simulink model "quadcopter_dynamic_model"  (R2016b)
settings: Solver=FixedStepAuto  StartTime=0.0  StopTime=30  FixedStep=0.001  MaxStep=0.004  RelTol=1e-3
PreLoadFcn:
  | init
undefined symbols (not defined in the file or in its folder): Data, Data_SL_Info, W, X, Y, Z
libraries: robotlib x7
settings Model: Creator=ADAM  LastModifiedBy=consti
settings SolverCC: ExtrapolationOrder=1
settings DataIOCC: MaxDataPoints=1  SaveFormat=Structure  SignalLoggingSaveFormat=ModelDataLogs  SaveOutput=off  SignalLogging=off  DSMLogging=off  SaveTime=off  OutputSaveName=model_out  SignalLoggingName=model_out
settings OptimizationCC: ExpressionDepthLimit=2147483647  LifeSpan=inf  SimCompilerOptimization=on
settings DebuggingCC: UnderspecifiedInitializationDetection=Classic  MergeDetectMultiDrivingBlocksExec=none  InheritedTsInSrcMsg=none  MultiTaskDSMMsg=warning  MultiTaskCondExecSysMsg=none  UnconnectedInputMsg=none  UnconnectedOutputMsg=none  UnconnectedLineMsg=none  StateNameClashWarn=warning  SFUnexpectedBacktrackingDiag=warning  SFNoUnconditionalDefaultTransitionDiag=warning  SFExecutionAtInitializationDiag=none
settings HardwareCC: ProdBitPerPointer=32  ProdBitPerSizeT=32  ProdBitPerPtrDiffT=32  ProdLargestAtomicFloat=None  ProdWordSize=32  ProdHWDeviceType=Generic->32-bit x86 compatible
settings ModelReferenceCC: UpdateModelReferenceTargets=IfOutOfDate  PropagateSignalLabelsOutOfModel=off
settings CodeAppCC: MaxIdLength=95
settings GRTTargetCC: TargetLangStandard=C89/C90 (ANSI)  GeneratePreprocessorConditionals=Disable all
settings ConfigComp: CovMetricSettings=dw  CovHtmlReporting=on  CovSaveCumulativeToWorkspaceVar=on  CovSaveSingleToWorkspaceVar=on  CovExternalEMLEnable=off  CovSFcnEnable=off

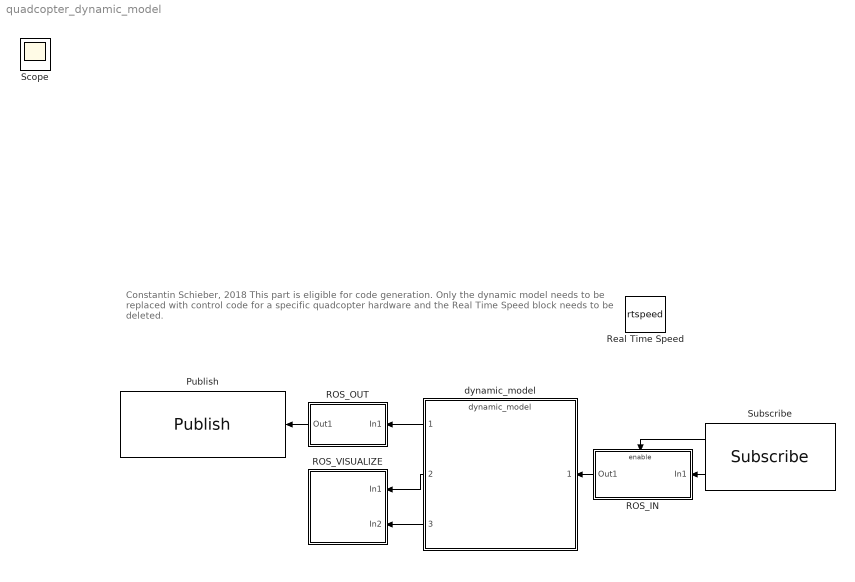
== system quadcopter_dynamic_model ==
  note: Constantin Schieber, 2018
      |
      | This part is eligible for code generation. Only the dynamic model needs to be replaced with control code
      | for a specific quadcopter hardware and the Real Time Speed block needs to be deleted.
  Publish : robotlib/Publish  SourceLibraryInfo=This block requires Robotics System Toolbox  topicSource=Specify your own  topic=/dyn_model_measurments  messageType=std_msgs/Float32MultiArray  messageQueueLength=1
  ROS_IN : Subsystem
  ROS_OUT : Subsystem
  ROS_VISUALIZE : Subsystem
  Real Time Speed : S-Function  FunctionName=rtspeed  Parameters=speed  SFunctionDeploymentMode=off  EnableBusSupport=off  mask(Simulink Realtime Synchronization){speed=1}
      mask prompts: speed "Simulation Speed (1 = realtime)"
      mask help: Slows down simulation to desired real time speed.
      mask Display:
      | ang=(0:0.0125:1)*2*pi;
      | xp=100*cos(ang);
      | yp=100*sin(ang);
      | plot(-145,-130,155,170,xp,yp,[0 0 70*sqrt(2)/2],[70 0 70*sqrt(2)/2],[-40 40 40 -40 -40],[150 150 120 120 150],[-15 -15],[120 98.5],[15 15],[120 98.5],[100*cos((45+9)/180*pi) 100*cos((45+9)/180*pi)+30 100*cos((45-9)/180*pi)+30 100*cos((45-9)/180*pi)],[100*sin((45+9)/180*pi) 100*sin((45+9)/180*pi)+30 100*sin((45-9)/180*pi)+30 100*sin((45-9)/180*pi)]);
  Subscribe : robotlib/Subscribe  SourceLibraryInfo=This block requires Robotics System Toolbox  topicSource=Specify your own  topic=/control_system_pwm  messageType=std_msgs/Float32MultiArray  sampleTime=-1  messageQueueLength=1
  dynamic_model : ModelReference  ModelNameDialog=dynamic_model  SimulationMode=Normal  ModelReferenceVersion=1.2329
  Scope : Scope
  wires:
  dynamic_model/2 -> ROS_VISUALIZE/1(In1)
  Subscribe/2 -> ROS_IN/1(In1)
  ROS_IN/1(Out1) -> dynamic_model/1
  dynamic_model/1 -> ROS_OUT/1(In1)
  ROS_OUT/1(Out1) -> Publish/1
  Subscribe/1 -> ROS_IN/Enable
  dynamic_model/3 -> ROS_VISUALIZE/2(In2)

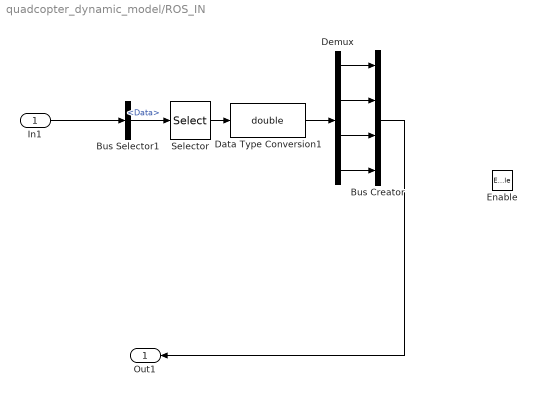
== system quadcopter_dynamic_model/ROS_IN ==
  In1 : Inport
  Enable : EnablePort
  Bus Creator : BusCreator  Inputs=4
  Bus Selector1 : BusSelector  OutputSignals=Data
  Data Type Conversion1 : DataTypeConversion  OutDataTypeStr=double
  Demux : Demux
  Selector : Selector  InputPortWidth=128  IndexOptions=Index vector (dialog)  Indices=[1 2 3 4]  OutputSizes=1
  Out1 : Outport
  wires:
  Data Type Conversion1/1 -> Demux/1
  Bus Creator/1 -> Out1/1
  In1/1 -> Bus Selector1/1
  Selector/1 -> Data Type Conversion1/1
  Bus Selector1/1 -> Selector/1  "<Data>"
  Demux/3 -> Bus Creator/3
  Demux/2 -> Bus Creator/2
  Demux/1 -> Bus Creator/1
  Demux/4 -> Bus Creator/4

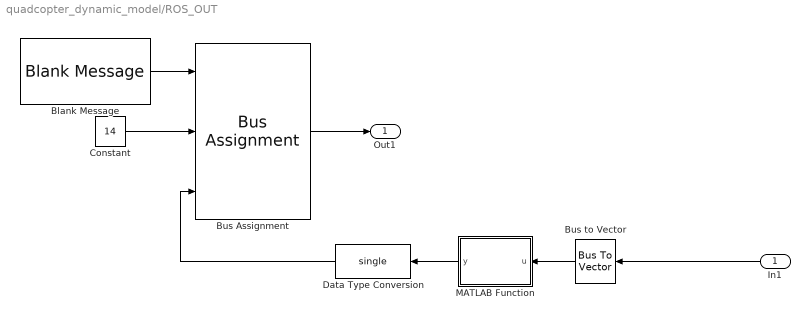
== system quadcopter_dynamic_model/ROS_OUT ==
  In1 : Inport
  Blank Message : robotlib/Blank Message  SourceLibraryInfo=This block requires Robotics System Toolbox  messageType=std_msgs/Float32MultiArray  SampleTime=inf
  Bus Assignment : BusAssignment  AssignedSignals=Data_SL_Info.CurrentLength,Data
  Bus to Vector : BusToVector
  Constant : Constant  Value=14  OutDataTypeStr=uint32
  Data Type Conversion : DataTypeConversion  OutDataTypeStr=single
  MATLAB Function : MATLAB Function  TreatAsAtomicUnit=on
  Out1 : Outport
  wires:
  Bus to Vector/1 -> MATLAB Function/1(u)
  Data Type Conversion/1 -> Bus Assignment/3
  Blank Message/1 -> Bus Assignment/1
  Bus Assignment/1 -> Out1/1
  Constant/1 -> Bus Assignment/2
  MATLAB Function/1(y) -> Data Type Conversion/1
  In1/1 -> Bus to Vector/1

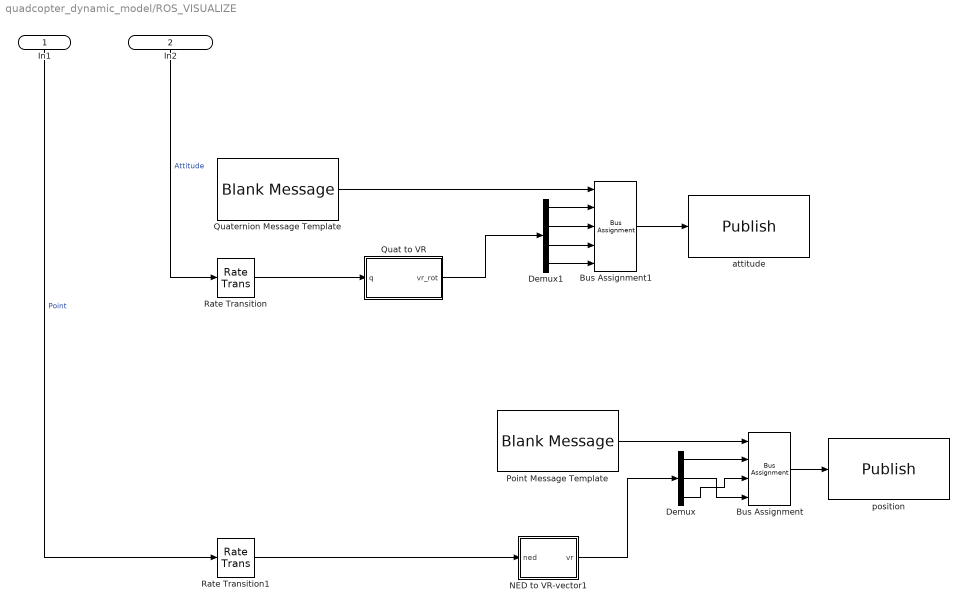
== system quadcopter_dynamic_model/ROS_VISUALIZE ==
  In1 : Inport
  In2 : Inport  Port=2
  Bus Assignment : BusAssignment  AssignedSignals=X,Y,Z
  Bus Assignment1 : BusAssignment  AssignedSignals=X,Y,Z,W
  Demux : Demux  Outputs=3
  Demux1 : Demux
  NED to VR-vector1 : Subsystem  mask(Converts NED to VR-vector){}
      mask help: [north east down] => [east up south]
  Point Message Template : robotlib/Blank Message  SourceLibraryInfo=This block requires Robotics System Toolbox  messageType=geometry_msgs/Point  SampleTime=inf
  Quat to VR : Subsystem  mask(Quaternion to VR-rotation){}
      mask help: Converts a normalized quaternion to a VR-rotation.
  Quaternion Message Template : robotlib/Blank Message  SourceLibraryInfo=This block requires Robotics System Toolbox  messageType=geometry_msgs/Quaternion  SampleTime=inf
  Rate Transition : RateTransition  Integrity=off  OutPortSampleTime=0.03
  Rate Transition1 : RateTransition  Integrity=off  OutPortSampleTime=0.03
  attitude : robotlib/Publish  SourceLibraryInfo=This block requires Robotics System Toolbox  topicSource=Specify your own  topic=/attitude_O  messageType=geometry_msgs/Quaternion  messageQueueLength=1
  position : robotlib/Publish  SourceLibraryInfo=This block requires Robotics System Toolbox  topicSource=Specify your own  topic=/position_O  messageType=geometry_msgs/Point  messageQueueLength=1
  wires:
  In1/1 -> Rate Transition1/1  "Point"
  Quaternion Message Template/1 -> Bus Assignment1/1
  Demux1/1 -> Bus Assignment1/2
  Demux1/2 -> Bus Assignment1/3
  Demux1/3 -> Bus Assignment1/4
  Demux1/4 -> Bus Assignment1/5
  Bus Assignment1/1 -> attitude/1
  Quat to VR/1(vr_rot) -> Demux1/1
  Point Message Template/1 -> Bus Assignment/1
  Bus Assignment/1 -> position/1
  NED to VR-vector1/1(vr) -> Demux/1
  Demux/1 -> Bus Assignment/2
  Demux/2 -> Bus Assignment/4
  Demux/3 -> Bus Assignment/3
  Rate Transition/1 -> Quat to VR/1(q)
  In2/1 -> Rate Transition/1  "Attitude"
  Rate Transition1/1 -> NED to VR-vector1/1(ned)

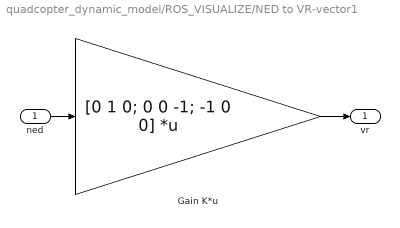
== system quadcopter_dynamic_model/ROS_VISUALIZE/NED to VR-vector1 ==
  ned : Inport
  Gain K*u : Gain  Gain=[0 1 0; 0 0 -1; -1 0 0]  Multiplication=Matrix(K*u)
  vr : Outport
  wires:
  Gain K*u/1 -> vr/1
  ned/1 -> Gain K*u/1

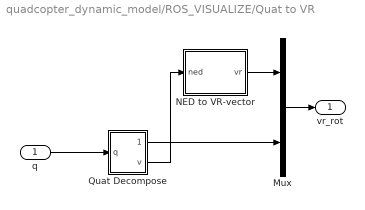
== system quadcopter_dynamic_model/ROS_VISUALIZE/Quat to VR ==
  q : Inport
  Mux : Mux  Inputs=2
  NED to VR-vector : Subsystem  mask(Converts NED to VR-vector){}
      mask help: [north east down] => [east up south]
  Quat Decompose : Subsystem  mask(Quaternion Decomposition){}
      mask help:
      | Decomposes a normalized Quaternion into
      | the rotation-vector v and the rotation-angle phi.
  vr_rot : Outport
  wires:
  q/1 -> Quat Decompose/1(q)
  Quat Decompose/2(v) -> NED to VR-vector/1(ned)
  NED to VR-vector/1(vr) -> Mux/1
  Quat Decompose/1(phi) -> Mux/2
  Mux/1 -> vr_rot/1

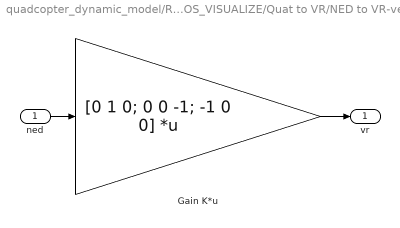
== system quadcopter_dynamic_model/ROS_VISUALIZE/Quat to VR/NED to VR-vector ==
  ned : Inport
  Gain K*u : Gain  Gain=[0 1 0; 0 0 -1; -1 0 0]  Multiplication=Matrix(K*u)
  vr : Outport
  wires:
  Gain K*u/1 -> vr/1
  ned/1 -> Gain K*u/1

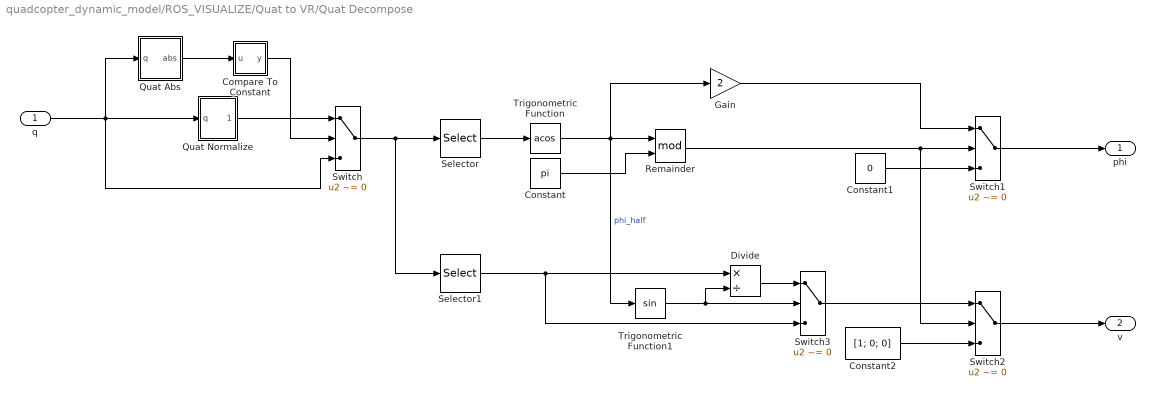
== system quadcopter_dynamic_model/ROS_VISUALIZE/Quat to VR/Quat Decompose ==
  q : Inport
  Compare To Constant : Subsystem  mask(Compare To Constant){relop=~=, const=1, OutDataTypeStr=uint8, ZeroCross=off}
      mask prompts: relop "Simulink:masks:Operator_MP"; const "Simulink:masks:ConstantValue_MP"; OutDataTypeStr "Simulink:masks:OutputDataType_MP"; ZeroCross "Simulink:masks:EnableZerocrossingDetection_MP"
      mask help: Simulink:masks:CompareToConstant_MD
      mask init:
      | blkName = gcb;
      | 
      | if strcmp(get_param(gcbh,'OutDataTypeStr'),'boolean')
      | 	setValue = 'boolean';
      | else
      | 	setValue = 'fixdt(0, 8)';
      | end
      | 
      | set_param([blkName,'/Compare'],'relop',relop, ...
      | 	'OutDataTypeStr', setValue, 'ZeroCross', ZeroCross);
      | 
      | str = [relop,' C']; %default
      | 
      | const_str = get_param(blkName, 'const');
      | 
      | if isempty(strfind(const_str, ' ')) && isempty(strfind(const_str, ','))
      |     % scalar or single expression
      |     if isempty(str2num(const_str))
      |         %expression
      |         str = [relop, ' ', const_str];
      |     elseif length(const) == 1
      |         str = [relop,' ',num2str(double(const))];
      |     end
      | end
      mask TypeOptions relop: == | ~= | < | <= | >= | >
      mask TypeOptions OutDataTypeStr: Simulink:masks:uint8 | Simulink:masks:boolean
      mask Callback ZeroCross: sl('zeroCrossEnable', gcbh);
      mask Display: disp(str)
  Constant : Constant  Value=pi  OutDataTypeStr=Inherit: Inherit via back propagation
  Constant1 : Constant  Value=0  VectorParams1D=off
  Constant2 : Constant  Value=[1; 0; 0]  VectorParams1D=off
  Divide : Product  Inputs=*/
  Gain : Gain  Gain=2
  Quat Abs : Subsystem  mask(Absolute value){}
      mask help: sqrt(q(1)^2+q(2)^2+q(3)^2+q(4)^2)
      mask init:
      | pos = get_param(gcb, 'Position');
      | width = pos(3) - pos(1); height = pos(4) - pos(2);
      | fontsize = get_param(gcb, 'fontsize');
      | if fontsize==-1, scale=1; else scale=fontsize/10; end
      mask Display: text(width/2-scale*8, (height/2-scale), '||q||')
  Quat Normalize : Subsystem  mask(Quaternion Normalize){}
      mask help:
      | if abs(q) ~= 0
      |     q_norm = q/sqrt(q(1)^2+q(2)^2+q(3)^2+q(4)^2)
      | else
      |     q_norm = [1; 0; 0; 0]
      |
      | Regrettably implemented in Simulink
      mask init:
      | pos = get_param(gcb, 'Position');
      | width = pos(3) - pos(1); height = pos(4) - pos(2);
      | fontsize = get_param(gcb, 'fontsize');
      | if fontsize==-1, scale=1; else scale=fontsize/10; end
      mask Display:
      | text(width/2-scale*3, (height/2+scale*10), 'q')
      | text(width/2-scale*8, (height/2-scale*6), '||q||')
      | plot([width/2-scale*10 width/2+scale*10], height/2*[1 1])
  Remainder : Math  Operator=mod  SaturateOnIntegerOverflow=on
  Selector : Selector  InputPortWidth=4  IndexOptions=Index vector (dialog)  Indices=[1]  OutputSizes=1
  Selector1 : Selector  InputPortWidth=4  IndexOptions=Index vector (dialog)  Indices=[2 3 4]  OutputSizes=1
  Switch{,1..3} (4 alike) : Switch  Criteria=u2 ~= 0
  Trigonometric Function : Trigonometry  Operator=acos
  Trigonometric Function1 : Trigonometry
  phi : Outport
  v : Outport  Port=2
  wires:
  q/1 -> Switch/3, Quat Abs/1(q), Quat Normalize/1(q)
  Quat Abs/1(abs) -> Compare To Constant/1(u)
  Compare To Constant/1(y) -> Switch/2
  Quat Normalize/1(q_norm) -> Switch/1
  Switch/1 -> Selector/1, Selector1/1
  Selector/1 -> Trigonometric Function/1
  Trigonometric Function/1 -> Remainder/1, Gain/1, Trigonometric Function1/1  "phi_half"
  Constant/1 -> Remainder/2
  Remainder/1 -> Switch1/2, Switch2/2
  Gain/1 -> Switch1/1
  Switch1/1 -> phi/1
  Switch2/1 -> v/1
  Constant1/1 -> Switch1/3
  Constant2/1 -> Switch2/3
  Trigonometric Function1/1 -> Switch3/2, Divide/2
  Switch3/1 -> Switch2/1
  Selector1/1 -> Divide/1, Switch3/3
  Divide/1 -> Switch3/1

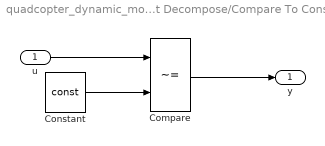
== system quadcopter_dynamic_model/ROS_VISUALIZE/Quat to VR/Quat Decompose/Compare To Constant ==
  u : Inport
  Compare : RelationalOperator  Operator=~=  OutDataTypeStr=fixdt(0, 8)  ZeroCross=off  RndMeth=Nearest  InputSameDT=on
  Constant : Constant  DisableCoverage=on  Value=const  OutDataTypeStr=Inherit: Inherit via back propagation
  y : Outport
  wires:
  Compare/1 -> y/1
  Constant/1 -> Compare/2
  u/1 -> Compare/1

== system quadcopter_dynamic_model/ROS_VISUALIZE/Quat to VR/Quat Decompose/Quat Abs ==
  q : Inport
  Euclidean_Norm : Subsystem
      mask help: Euclidean Norm
      mask Help: Euclidean Norm
      mask Display: disp('||.||')
  abs : Outport
  wires:
  q/1 -> Euclidean_Norm/1(u)
  Euclidean_Norm/1(||u||) -> abs/1

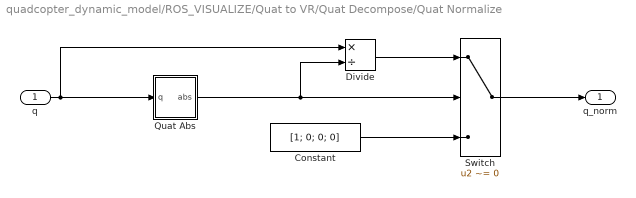
== system quadcopter_dynamic_model/ROS_VISUALIZE/Quat to VR/Quat Decompose/Quat Normalize ==
  q : Inport
  Constant : Constant  Value=[1; 0; 0; 0]  VectorParams1D=off  OutDataTypeStr=Inherit: Inherit via back propagation
  Divide : Product  Inputs=*/  OutMin=-1.5  OutMax=1.5  OutDataTypeStr=Inherit: Same as first input
  Quat Abs : Subsystem  mask(Absolute value){}
      mask help: sqrt(q(1)^2+q(2)^2+q(3)^2+q(4)^2)
      mask init:
      | pos = get_param(gcb, 'Position');
      | width = pos(3) - pos(1); height = pos(4) - pos(2);
      | fontsize = get_param(gcb, 'fontsize');
      | if fontsize==-1, scale=1; else scale=fontsize/10; end
      mask Display: text(width/2-scale*8, (height/2-scale), '||q||')
  Switch : Switch  Criteria=u2 ~= 0
  q_norm : Outport
  wires:
  Constant/1 -> Switch/3
  Divide/1 -> Switch/1
  Quat Abs/1(abs) -> Divide/2, Switch/2
  q/1 -> Divide/1, Quat Abs/1(q)
  Switch/1 -> q_norm/1

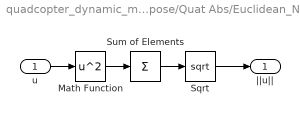
== system quadcopter_dynamic_model/ROS_VISUALIZE/Quat to VR/Quat Decompose/Quat Abs/Euclidean_Norm ==
  u : Inport
  Math Function : Math  Operator=square  SaturateOnIntegerOverflow=on
  Sqrt : Sqrt  SaturateOnIntegerOverflow=on
  Sum of Elements : Sum  Inputs=+
  ||u|| : Outport
  wires:
  Sqrt/1 -> ||u||/1
  Sum of Elements/1 -> Sqrt/1
  Math Function/1 -> Sum of Elements/1
  u/1 -> Math Function/1

== system quadcopter_dynamic_model/ROS_VISUALIZE/Quat to VR/Quat Decompose/Quat Normalize/Quat Abs ==
  q : Inport
  Euclidean_Norm : Subsystem
      mask help: Euclidean Norm
      mask Help: Euclidean Norm
      mask Display: disp('||.||')
  abs : Outport
  wires:
  q/1 -> Euclidean_Norm/1(u)
  Euclidean_Norm/1(||u||) -> abs/1

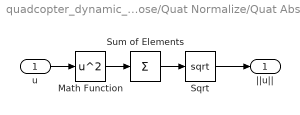
== system quadcopter_dynamic_model/ROS_VISUALIZE/Quat to VR/Quat Decompose/Quat Normalize/Quat Abs/Euclidean_Norm ==
  u : Inport
  Math Function : Math  Operator=square  SaturateOnIntegerOverflow=on
  Sqrt : Sqrt  SaturateOnIntegerOverflow=on
  Sum of Elements : Sum  Inputs=+
  ||u|| : Outport
  wires:
  Sqrt/1 -> ||u||/1
  Sum of Elements/1 -> Sqrt/1
  Math Function/1 -> Sum of Elements/1
  u/1 -> Math Function/1

== matlab function quadcopter_dynamic_model/ROS_OUT/MATLAB Function ==
  data: u input; y output
function y = fcn(u)


y = zeros(1,128);
for i = 1:14
    y(i) = u(i);
end
end
